simulink model "battery_char"  (R2019b)
settings: Solver=VariableStepAuto  StartTime=0.0  StopTime=tsimulation  RelTol=1e-3
values from neighbouring files (symbols this model uses):
  C = Cbat*Nbp*3600    (= 37440)    [demoEPS.m]    (also in demoEPS_R2019a.m; demoEPS_v1.m; demoEPS_v1a.m; demoEPS_v1test.m)
  eff_bc = 0.9    [testsim.m]
  iCharge = 8    [testsim.m]
  Nbs = math.ceil(Vbusmin/Vbatmin)    [calc_mass_EPS.m]    (also in demoEPS.m = 4; demoEPS_R2019a.m = 4; demoEPS_v1.m = 4; demoEPS_v1a.m = 4)
  SOC_0 = 0    [testsim.m]
libraries: simulink x1
settings Model: Creator=Ricardo  LastModifiedBy=Ricardo

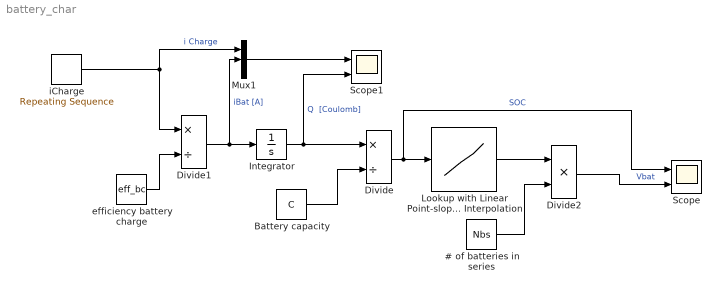
== system battery_char ==
  # of batteries in series : Constant  Value=Nbs
  Battery capacity : Constant  Value=C
  Divide : Product  Inputs=*/
  Divide1 : Product  Inputs=*/
  Divide2 : Product  Inputs=**
  Integrator : Integrator  InitialCondition=SOC_0
  Lookup with Linear Point-slope Interpolation : Lookup_n-D  NumberOfTableDimensions=1  BreakpointsForDimension1=[0,0.05,0.09,0.18,0.37,0.51,0.6,0.74,0.84,0.95,1]  Table=[2.75,2.9,3.4,3.5,3.6,3.7,3.8,3.9,4,4.1,4.2]  InternalRulePriority=Speed  RndMeth=Simplest  InputSameDT=on
  Mux1 : Mux  Inputs=3
  Scope : Scope  NumInputPorts=2
  Scope1 : Scope  NumInputPorts=2
  efficiency battery charge : Constant  Value=eff_bc
  iCharge : simulink/Sources/Repeating Sequence  rep_seq_t=[0 100 100.1 110]  rep_seq_y=[iCharge iCharge 0 0]
  wires:
  Mux1/1 -> Scope1/1
  Divide1/1 -> Mux1/2, Integrator/1  "iBat [A]"
  efficiency battery charge/1 -> Divide1/2
  # of batteries in series/1 -> Divide2/2
  Divide2/1 -> Scope/2  "Vbat"
  Integrator/1 -> Scope1/2, Divide/1  "Q  [Coulomb]"
  Battery capacity/1 -> Divide/2
  iCharge/1 -> Divide1/1, Mux1/1  "i Charge"
  Divide/1 -> Lookup with Linear Point-slope Interpolation/1, Scope/1  "SOC"
  Lookup with Linear Point-slope Interpolation/1 -> Divide2/1
